simulink model "AttitudeControl"  (R2020b)
settings: Solver=ode45  StartTime=0.0  StopTime=2000  RelTol=1e-3  EnableMultiTasking=on
libraries: simulink_extras x4, simulink x4
settings Model: Creator=G_C  LastModifiedBy=alam
settings DataIOCC: LimitDataPoints=on  SaveFormat=Array  ReturnWorkspaceOutputs=off
settings OptimizationCC: LifeSpan=inf
settings DebuggingCC: SolverPrmCheckMsg=warning  SFUnexpectedBacktrackingDiag=warning  SFNoUnconditionalDefaultTransitionDiag=warning  SFExecutionAtInitializationDiag=none  ArithmeticOperatorsInVariantConditions=warning
settings HardwareCC: ProdBitPerPointer=32  ProdBitPerSizeT=32  ProdBitPerPtrDiffT=32  ProdLargestAtomicFloat=None  ProdIntDivRoundTo=Undefined  ProdEndianess=Unspecified  ProdWordSize=32  ProdHWDeviceType=32-bit Generic
settings ModelReferenceCC: PropagateSignalLabelsOutOfModel=off
settings SFSimCC: SimUseLocalCustomCode=off  CustomCodeUndefinedFunction=UseInterfaceOnly
settings RTWCC: RTWUseLocalCustomCode=off
settings CodeAppCC: StateflowObjectComments=on
settings GRTTargetCC: TargetLangStandard=C89/C90 (ANSI)
settings ConfigComp: CovMetricSettings=dw  CovSaveCumulativeToWorkspaceVar=on  CovSaveSingleToWorkspaceVar=on  CovExternalEMLEnable=off  CovSFcnEnable=off

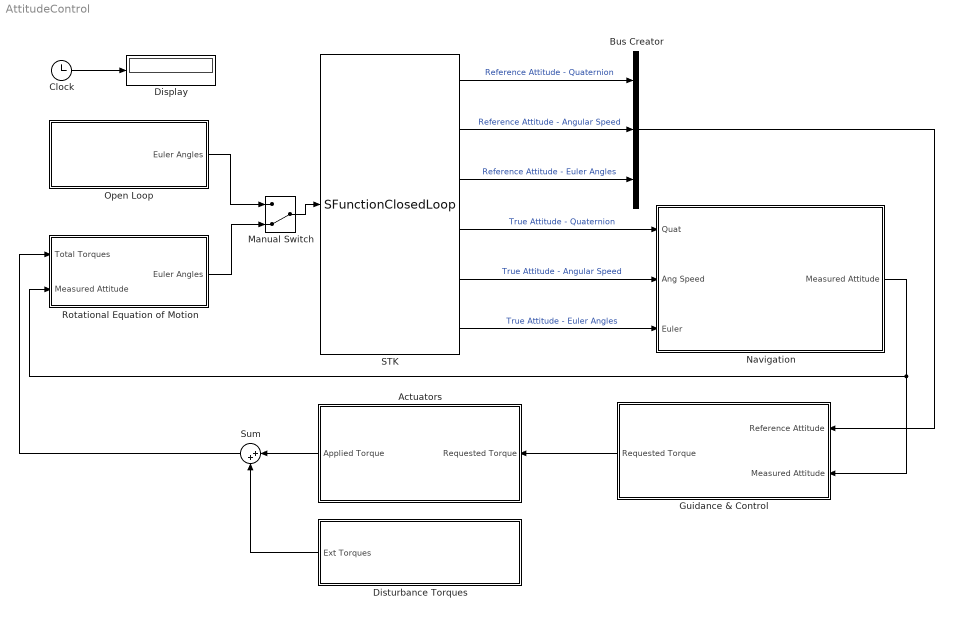
== system AttitudeControl ==
  Actuators : Subsystem
  Bus Creator : BusCreator  Inputs=3
  Clock : Clock
  Display : Display
  Disturbance Torques : Subsystem
  Guidance & Control : Subsystem
  Manual Switch : ManualSwitch  CurrentSetting=0
  Navigation : Subsystem
  Open Loop : Subsystem
  Rotational Equation of Motion : Subsystem
  STK : M-S-Function  InitFcn=|  FunctionName=SFunctionClosedLoop
      | close all
      | clear all
      | clc
      | 
      | %create a new instance of STK12
      | uiapp = actxserver('STK12.Application');
      | uiapp.visible = 1;
      | 
      | %get the object model root for STK12, IAgStkObjectRoot 
      | root = uiapp.Personality2;
      | 
      | root.LoadScenario('C:\SimulinkAttitudeControlLoop\Attitude_Control.sc');
      | objSat=root.GetObjectFromPath('/Satellite/True');
      | objRef=root.GetObjectFromPath('/Satellite/Reference');
      | 
      | %reset the scenario
      | root.ExecuteCommand('Animate * Reset');
      | 
      | %store the STK parameters
      | stkParams = cell(4,1);
      | stkParams{1} = uiapp;
      | stkParams{2} = root;
      | stkParams{3} = objSat;
      | stkParams{4} = objRef;
      | 
      | set_param(gcb, 'UserData', stkParams);
      | 
      | root.ExecuteCommand('SetUnits / EpSec');
      | root.UnitPreferences.SetCurrentUnit('DateFormat', 'EpSec');
  Sum : Sum  Inputs=|++
  wires:
  Clock/1 -> Display/1
  Actuators/1(Applied Torque) -> Sum/1
  Disturbance Torques/1(Ext Torques) -> Sum/2
  Open Loop/1(Euler Angles) -> Manual Switch/1
  Manual Switch/1 -> STK/1
  STK/3 -> Bus Creator/3  "Reference Attitude - Euler Angles"
  STK/4 -> Navigation/1(Quat)  "True Attitude - Quaternion"
  STK/1 -> Bus Creator/1  "Reference Attitude - Quaternion"
  STK/2 -> Bus Creator/2  "Reference Attitude - Angular Speed"
  STK/5 -> Navigation/2(Ang Speed)  "True Attitude - Angular Speed"
  STK/6 -> Navigation/3(Euler)  "True Attitude - Euler Angles"
  Guidance & Control/1(Requested Torque) -> Actuators/1(Requested Torque)
  Bus Creator/1 -> Guidance & Control/1(Reference Attitude)
  Sum/1 -> Rotational Equation of Motion/1(Total Torques)
  Rotational Equation of Motion/1(Euler Angles) -> Manual Switch/2
  Navigation/1(Measured Attitude) -> Rotational Equation of Motion/2(Measured Attitude), Guidance & Control/2(Measured Attitude)

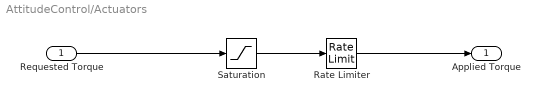
== system AttitudeControl/Actuators ==
  Requested Torque : Inport
  Rate Limiter : RateLimiter  RisingSlewLimit=10  FallingSlewLimit=-10
  Saturation : Saturate  UpperLimit=50  LowerLimit=-50
  Applied Torque : Outport
  wires:
  Requested Torque/1 -> Saturation/1
  Saturation/1 -> Rate Limiter/1
  Rate Limiter/1 -> Applied Torque/1

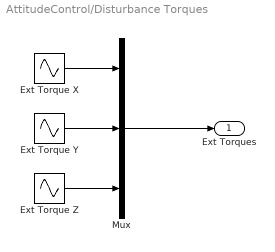
== system AttitudeControl/Disturbance Torques ==
  Ext Torque X : Sin  Amplitude=1e-6  Frequency=0.0021  SampleTime=0
  Ext Torque Y : Sin  Amplitude=1e-6  Frequency=0.0021  Phase=100  SampleTime=0
  Ext Torque Z : Sin  Amplitude=1e-6  Frequency=0.0021  Phase=50  SampleTime=0
  Mux : Mux  Inputs=3
  Ext Torques : Outport
  wires:
  Ext Torque X/1 -> Mux/1
  Ext Torque Y/1 -> Mux/2
  Ext Torque Z/1 -> Mux/3
  Mux/1 -> Ext Torques/1

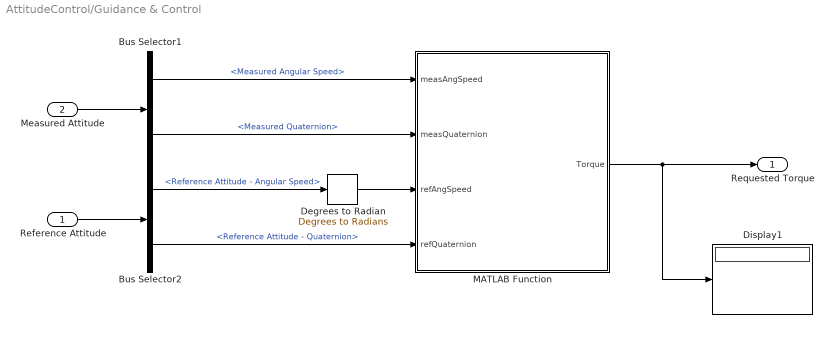
== system AttitudeControl/Guidance & Control ==
  Reference Attitude : Inport
  Measured Attitude : Inport  Port=2
  Bus Selector1 : BusSelector  OutputSignals=Measured Angular Speed,Measured Quaternion
  Bus Selector2 : BusSelector  OutputSignals=Reference Attitude - Angular Speed,Reference Attitude - Quaternion
  Degrees to Radian : simulink_extras/Transformations/Degrees to Radians
  Display1 : Display
  MATLAB Function : MATLAB Function  TreatAsAtomicUnit=on
  Requested Torque : Outport
  wires:
  Reference Attitude/1 -> Bus Selector2/1
  Measured Attitude/1 -> Bus Selector1/1
  Bus Selector1/1 -> MATLAB Function/1(measAngSpeed)  "<Measured Angular Speed>"
  Bus Selector2/1 -> Degrees to Radian/1  "<Reference Attitude - Angular Speed>"
  MATLAB Function/1(Torque) -> Display1/1, Requested Torque/1
  Bus Selector2/2 -> MATLAB Function/4(refQuaternion)  "<Reference Attitude - Quaternion>"
  Bus Selector1/2 -> MATLAB Function/2(measQuaternion)  "<Measured Quaternion>"
  Degrees to Radian/1 -> MATLAB Function/3(refAngSpeed)

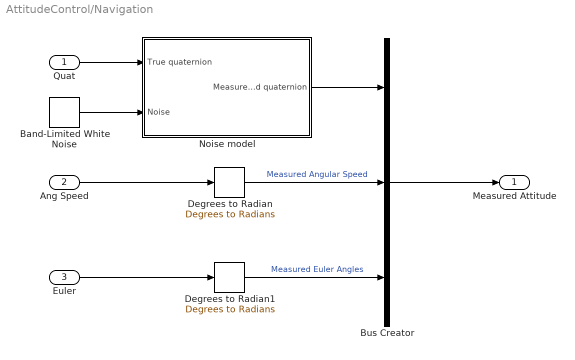
== system AttitudeControl/Navigation ==
  Quat : Inport
  Ang Speed : Inport  Port=2
  Euler : Inport  Port=3
  Band-Limited White Noise : simulink/Sources/Band-Limited White Noise  Cov=[0]  Ts=1  seed=[23341]
  Bus Creator : BusCreator  Inputs=3
  Degrees to Radian : simulink_extras/Transformations/Degrees to Radians
  Degrees to Radian1 : simulink_extras/Transformations/Degrees to Radians
  Noise model : Subsystem
  Measured Attitude : Outport
  wires:
  Ang Speed/1 -> Degrees to Radian/1
  Bus Creator/1 -> Measured Attitude/1
  Euler/1 -> Degrees to Radian1/1
  Degrees to Radian/1 -> Bus Creator/2  "Measured Angular Speed"
  Quat/1 -> Noise model/1(True quaternion)
  Noise model/1(Measured quaternion) -> Bus Creator/1
  Band-Limited White Noise/1 -> Noise model/2(Noise)
  Degrees to Radian1/1 -> Bus Creator/3  "Measured Euler Angles"

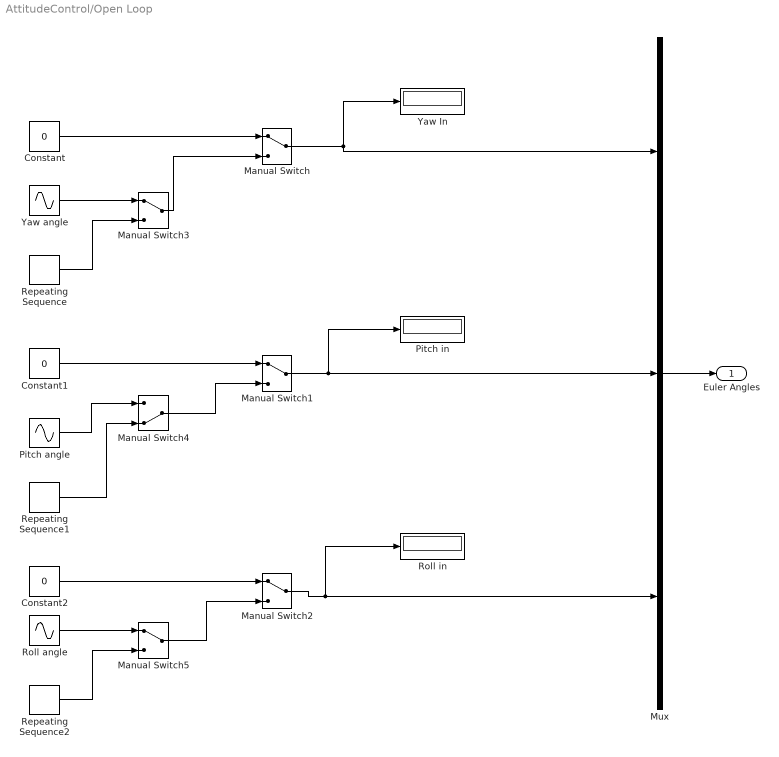
== system AttitudeControl/Open Loop ==
  Constant : Constant  Value=0
  Constant1 : Constant  Value=0
  Constant2 : Constant  Value=0
  Manual Switch{,1..3,5} (5 alike) : ManualSwitch
  Manual Switch4 : ManualSwitch  CurrentSetting=0
  Mux : Mux  Inputs=3
  Pitch angle : Sin  Amplitude=90  Frequency=0.016  Phase=9  SampleTime=0
  Pitch in : Display
  Repeating Sequence : simulink/Sources/Repeating Sequence  rep_seq_t=[0 60]  rep_seq_y=[0 360]
  Repeating Sequence1 : simulink/Sources/Repeating Sequence  rep_seq_t=[0 60]  rep_seq_y=[0 360]
  Repeating Sequence2 : simulink/Sources/Repeating Sequence  rep_seq_t=[0 60]  rep_seq_y=[0 360]
  Roll angle : Sin  Amplitude=90  Frequency=0.1  Phase=60  SampleTime=0
  Roll in : Display
  Yaw In : Display
  Yaw angle : Sin  Amplitude=90  Frequency=0.01  SampleTime=0
  Euler Angles : Outport
  wires:
  Constant/1 -> Manual Switch/1
  Manual Switch/1 -> Yaw In/1, Mux/1
  Constant1/1 -> Manual Switch1/1
  Manual Switch1/1 -> Mux/2, Pitch in/1
  Constant2/1 -> Manual Switch2/1
  Manual Switch2/1 -> Mux/3, Roll in/1
  Mux/1 -> Euler Angles/1
  Yaw angle/1 -> Manual Switch3/1
  Repeating Sequence/1 -> Manual Switch3/2
  Manual Switch3/1 -> Manual Switch/2
  Pitch angle/1 -> Manual Switch4/1
  Repeating Sequence1/1 -> Manual Switch4/2
  Manual Switch4/1 -> Manual Switch1/2
  Roll angle/1 -> Manual Switch5/1
  Repeating Sequence2/1 -> Manual Switch5/2
  Manual Switch5/1 -> Manual Switch2/2

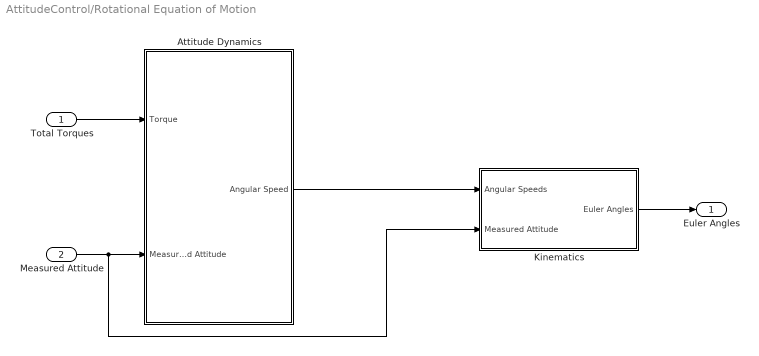
== system AttitudeControl/Rotational Equation of Motion ==
  Total Torques : Inport
  Measured Attitude : Inport  Port=2
  Attitude Dynamics : Subsystem
  Kinematics : Subsystem
  Euler Angles : Outport
  wires:
  Total Torques/1 -> Attitude Dynamics/1(Torque)
  Measured Attitude/1 -> Kinematics/2(Measured Attitude), Attitude Dynamics/2(" Measured Attitude")
  Attitude Dynamics/1(Angular Speed) -> Kinematics/1(Angular Speeds)
  Kinematics/1(Euler Angles) -> Euler Angles/1

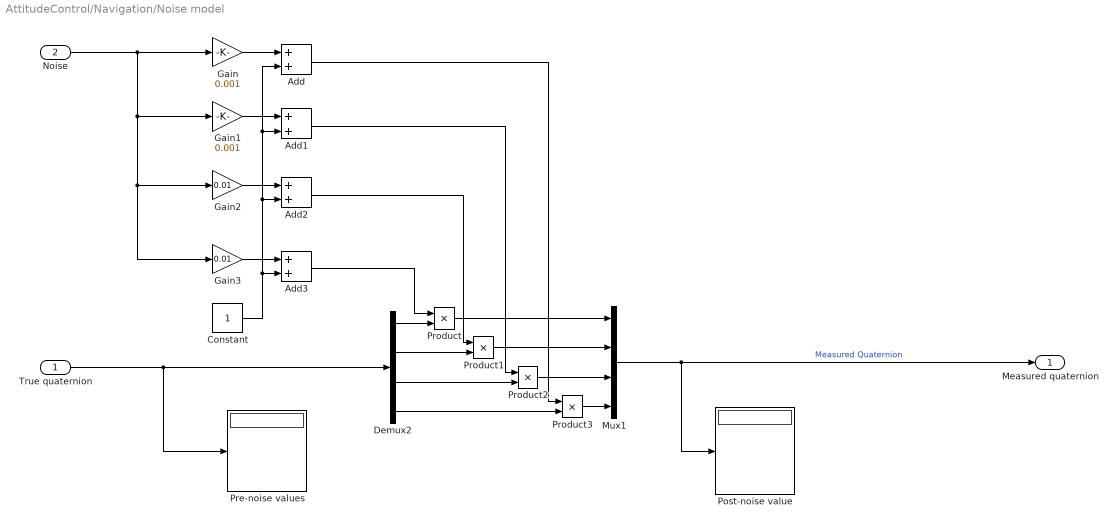
== system AttitudeControl/Navigation/Noise model ==
  True quaternion : Inport
  Noise : Inport  Port=2
  Add{,1..3} (4 alike) : Sum
  Constant : Constant
  Demux2 : Demux
  Gain : Gain  Gain=0.001
  Gain1 : Gain  Gain=0.001
  Gain2 : Gain  Gain=0.01
  Gain3 : Gain  Gain=0.01
  Mux1 : Mux
  Post-noise value : Display
  Pre-noise values : Display
  Product{,1..3} (4 alike) : Product
  Measured quaternion : Outport
  wires:
  True quaternion/1 -> Pre-noise values/1, Demux2/1
  Demux2/1 -> Product/2
  Demux2/2 -> Product1/2
  Demux2/3 -> Product2/2
  Demux2/4 -> Product3/2
  Mux1/1 -> Post-noise value/1, Measured quaternion/1  "Measured Quaternion"
  Product/1 -> Mux1/1
  Product1/1 -> Mux1/2
  Product2/1 -> Mux1/3
  Product3/1 -> Mux1/4
  Noise/1 -> Gain3/1, Gain2/1, Gain1/1, Gain/1
  Add3/1 -> Product/1
  Add2/1 -> Product1/1
  Add1/1 -> Product2/1
  Add/1 -> Product3/1
  Gain3/1 -> Add3/1
  Gain2/1 -> Add2/1
  Gain1/1 -> Add1/1
  Gain/1 -> Add/1
  Constant/1 -> Add2/2, Add1/2, Add/2, Add3/2

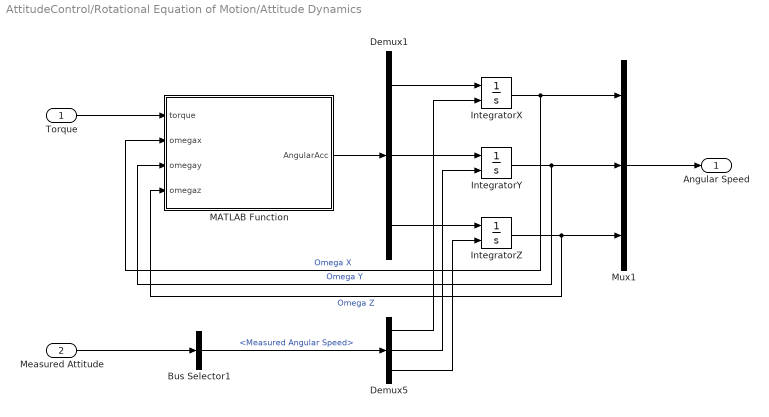
== system AttitudeControl/Rotational Equation of Motion/Attitude Dynamics ==
  Torque : Inport
  " Measured Attitude" : Inport  Port=2
  Bus Selector1 : BusSelector  OutputSignals=Measured Angular Speed
  Demux1 : Demux  Outputs=3
  Demux5 : Demux  Outputs=3
  IntegratorX : Integrator  InitialConditionSource=external
  IntegratorY : Integrator  InitialConditionSource=external
  IntegratorZ : Integrator  InitialConditionSource=external
  MATLAB Function : MATLAB Function  TreatAsAtomicUnit=on
  Mux1 : Mux  Inputs=3
  Angular Speed : Outport
  wires:
  " Measured Attitude"/1 -> Bus Selector1/1
  Bus Selector1/1 -> Demux5/1  "<Measured Angular Speed>"
  MATLAB Function/1(AngularAcc) -> Demux1/1
  Demux1/1 -> IntegratorX/1
  Demux1/2 -> IntegratorY/1
  Demux1/3 -> IntegratorZ/1
  IntegratorX/1 -> MATLAB Function/2(omegax), Mux1/1  "Omega X"
  IntegratorY/1 -> MATLAB Function/3(omegay), Mux1/2  "Omega Y"
  IntegratorZ/1 -> MATLAB Function/4(omegaz), Mux1/3  "Omega Z"
  Mux1/1 -> Angular Speed/1
  Torque/1 -> MATLAB Function/1(torque)
  Demux5/1 -> IntegratorX/2
  Demux5/2 -> IntegratorY/2
  Demux5/3 -> IntegratorZ/2

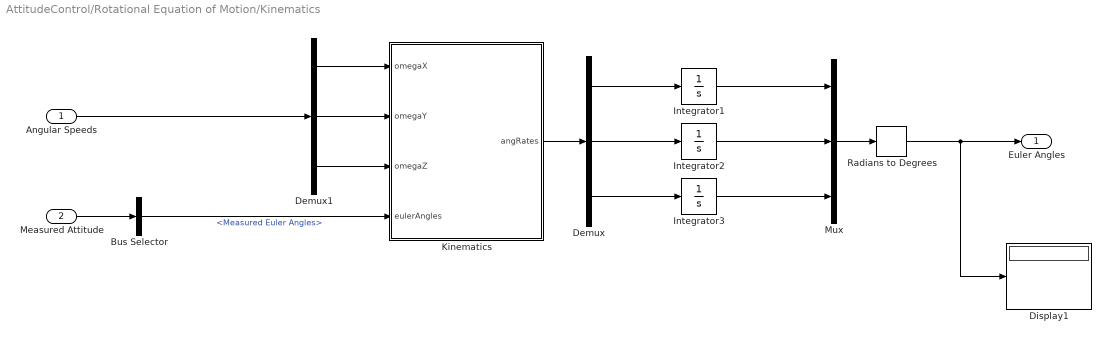
== system AttitudeControl/Rotational Equation of Motion/Kinematics ==
  Angular Speeds : Inport
  Measured Attitude : Inport  Port=2
  Bus Selector : BusSelector  OutputSignals=Measured Euler Angles
  Demux : Demux  Outputs=3
  Demux1 : Demux  Outputs=3
  Display1 : Display
  Integrator1 : Integrator
  Integrator2 : Integrator
  Integrator3 : Integrator
  Kinematics : MATLAB Function  TreatAsAtomicUnit=on
  Mux : Mux  Inputs=3
  Radians to Degrees : simulink_extras/Transformations/Radians to Degrees
  Euler Angles : Outport
  wires:
  Angular Speeds/1 -> Demux1/1
  Integrator1/1 -> Mux/1
  Integrator2/1 -> Mux/2
  Integrator3/1 -> Mux/3
  Measured Attitude/1 -> Bus Selector/1
  Bus Selector/1 -> Kinematics/4(eulerAngles)  "<Measured Euler Angles>"
  Kinematics/1(angRates) -> Demux/1
  Demux/1 -> Integrator1/1
  Demux/2 -> Integrator2/1
  Demux/3 -> Integrator3/1
  Mux/1 -> Radians to Degrees/1
  Demux1/2 -> Kinematics/2(omegaY)
  Demux1/3 -> Kinematics/3(omegaZ)
  Demux1/1 -> Kinematics/1(omegaX)
  Radians to Degrees/1 -> Display1/1, Euler Angles/1

== matlab function AttitudeControl/Guidance & Control/MATLAB Function ==
  data: measAngSpeed input; measQuaternion input; refAngSpeed input; Torque output; refQuaternion input
function Torque = TorqueController(measAngSpeed, measQuaternion, refAngSpeed, refQuaternion)

q = measQuaternion;
q1 = refQuaternion(1);
q2 = refQuaternion(2);
q3 = refQuaternion(3);
q4 = refQuaternion(4);

qE = qError(q1, q2, q3, q4, q);

wE = measAngSpeed - refAngSpeed;

%KP = ones(3,1)*40;
%KD = ones(3,1)*400;
KP = ones(3,1)*80;
KD = ones(3,1)*800;

Torque = -(sign(qE(4))*qE(1:3)'.*KP' + wE'.*KD');


function qE = qError(q1, q2, q3, q4, q)
q =  [q(4);q(1:3)];
qE = [q4 q1 q2 q3;-q1 q4 q3 -q2;-q2 -q3 q4 q1;-q3 q2 -q1 q4]*q;
qE = [qE(2:4);qE(1)];


% function Torque = TorqueController(measAngSpeed, refAngSpeed)
% 
% Ixx = 4500;
% Iyy = 4500;
% Izz = 4500;
% 
% omegax = measAngSpeed(1);
% omegay = measAngSpeed(2);
% omegaz = measAngSpeed(3);
% 
% omegaRefx = refAngSpeed(1);
% omegaRefy = refAngSpeed(2);
% omegaRefz = refAngSpeed(3);
% 
% Kp1 = 100;
% Kp2 = 100;
% Kp3 = 100;
% 
% Tx = -(Iyy - Izz)*omegay*omegaz - Kp1*(omegax - omegaRefx);
% Ty = -(Izz - Ixx)*omegaz*omegax - Kp2*(omegay - omegaRefy);
% Tz = -(Ixx - Iyy)*omegax*omegay - Kp3*(omegaz - omegaRefz);
% 
% 
% Torque = [Tx; Ty; Tz];

== matlab function AttitudeControl/Rotational Equation of Motion/Attitude Dynamics/MATLAB Function ==
  data: torque input; AngularAcc output; omegax input; omegay input; omegaz input
function AngularAcc = Euler(torque, omegax, omegay, omegaz)
% this function aoutputs
torquex = torque(1);
torquey = torque(2);
torquez = torque(3);

% satellite inertia
Ix = 450;
Iy = 450;
Iz = 350;

omegaDotx = (1/Ix)*(torquex + (Iy-Iz)*omegay*omegaz);
omegaDoty = (1/Iy)*(torquey + (Iz-Ix)*omegaz*omegax);
omegaDotz = (1/Iz)*(torquez + (Ix-Iy)*omegax*omegay);


AngularAcc = [omegaDotx; omegaDoty; omegaDotz];

== matlab function AttitudeControl/Rotational Equation of Motion/Kinematics/Kinematics ==
  data: omegaX input; omegaY input; omegaZ input; angRates output; eulerAngles input
function angRates = fcn(omegaX,omegaY,omegaZ,eulerAngles)



% omegaX = (3.14159/180)*omegaX;
% omegaY = (3.14159/180)*omegaY;
% omegaZ = (3.14159/180)*omegaZ;
phi = eulerAngles(1);
theta = eulerAngles(2);
psi = eulerAngles(3);


phiDot = sin(psi)*sec(theta)*omegaY + cos(psi)*sec(theta)*omegaZ;
thetaDot = cos(psi)*omegaY - sin(psi)*omegaZ;
psiDot = omegaX + sin(psi)*tan(theta)*omegaY + cos(psi)*tan(theta)*omegaZ;
angRates = [phiDot; thetaDot; psiDot];
